simulink model "ADS"  (R2022a)
settings: Solver=VariableStepAuto  StartTime=0.0  StopTime=10.0  RelTol=1e-3
values from neighbouring files (symbols this model uses):
  GyroB = deg2rad(3/3600) * randn * ones(3,1)    [backend.m]
  T = 0.1    [ADS.m]    (also in backend.m)
undefined symbols (not defined in the file or in its folder): magnitude
libraries: commchan3 x1
settings Model: Creator=emmamarsden  LastModifiedBy=emmamarsden

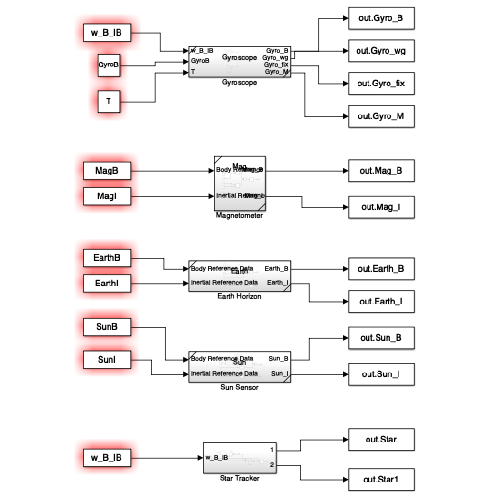
[thumbnail: Simulink's stored preview of the top-level diagram]
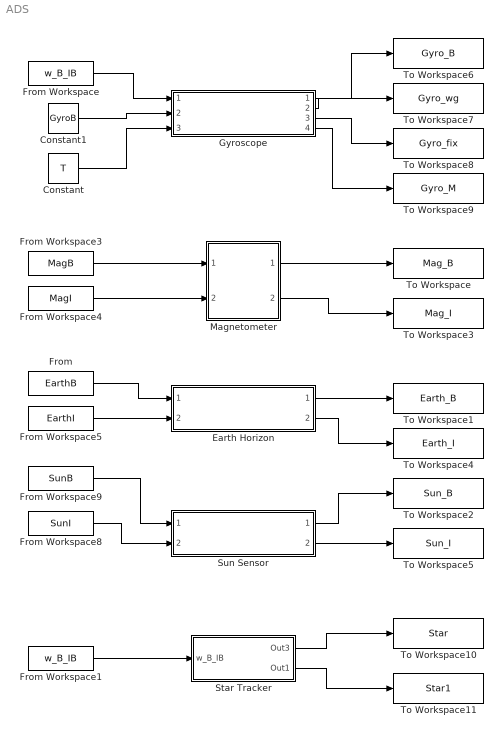
== system ADS ==
  Constant : Constant  Value=T
  Constant1 : Constant  Value=GyroB
  Earth Horizon : Subsystem  ReferencedSubsystem=Earth
  From : FromWorkspace  VariableName=EarthB  SampleTime=-1  ZeroCross=off
  From Workspace : FromWorkspace  VariableName=w_B_IB
  From Workspace1 : FromWorkspace  VariableName=w_B_IB
  From Workspace3 : FromWorkspace  VariableName=MagB
  From Workspace4 : FromWorkspace  VariableName=MagI
  From Workspace5 : FromWorkspace  VariableName=EarthI  ZeroCross=off
  From Workspace8 : FromWorkspace  VariableName=SunI
  From Workspace9 : FromWorkspace  VariableName=SunB
  Gyroscope : Subsystem  ReferencedSubsystem=Gyroscope
  Magnetometer : Subsystem  ReferencedSubsystem=Mag
  Star Tracker : Subsystem
  Sun Sensor : Subsystem  ReferencedSubsystem=Sun
  To Workspace : ToWorkspace  VariableName=Mag_B  SampleTime=-1
  To Workspace1 : ToWorkspace  VariableName=Earth_B  SampleTime=-1
  To Workspace10 : ToWorkspace  VariableName=Star  SaveFormat=Timeseries  SampleTime=-1
  To Workspace11 : ToWorkspace  VariableName=Star1  SaveFormat=Timeseries  SampleTime=-1
  To Workspace2 : ToWorkspace  VariableName=Sun_B  SaveFormat=Structure  SampleTime=-1
  To Workspace3 : ToWorkspace  VariableName=Mag_I  SampleTime=-1
  To Workspace4 : ToWorkspace  VariableName=Earth_I  SampleTime=-1
  To Workspace5 : ToWorkspace  VariableName=Sun_I  SaveFormat=Structure  SampleTime=-1
  To Workspace6 : ToWorkspace  VariableName=Gyro_B  SampleTime=-1
  To Workspace7 : ToWorkspace  VariableName=Gyro_wg  SampleTime=-1
  To Workspace8 : ToWorkspace  VariableName=Gyro_fix  SampleTime=-1
  To Workspace9 : ToWorkspace  VariableName=Gyro_M  SampleTime=-1
  wires:
  From Workspace5/1 -> Earth Horizon/2
  From Workspace4/1 -> Magnetometer/2
  From Workspace3/1 -> Magnetometer/1
  Magnetometer/1 -> To Workspace/1
  Magnetometer/2 -> To Workspace3/1
  Earth Horizon/1 -> To Workspace1/1
  Earth Horizon/2 -> To Workspace4/1
  From Workspace9/1 -> Sun Sensor/1
  From Workspace8/1 -> Sun Sensor/2
  From/1 -> Earth Horizon/1
  Sun Sensor/2 -> To Workspace5/1
  Sun Sensor/1 -> To Workspace2/1
  Constant1/1 -> Gyroscope/2
  From Workspace/1 -> Gyroscope/1
  Gyroscope/1 -> To Workspace6/1
  Gyroscope/2 -> To Workspace7/1
  Gyroscope/3 -> To Workspace8/1
  Gyroscope/4 -> To Workspace9/1
  Constant/1 -> Gyroscope/3
  From Workspace1/1 -> Star Tracker/1(w_B_IB)
  Star Tracker/1(Out3) -> To Workspace10/1
  Star Tracker/2(Out1) -> To Workspace11/1

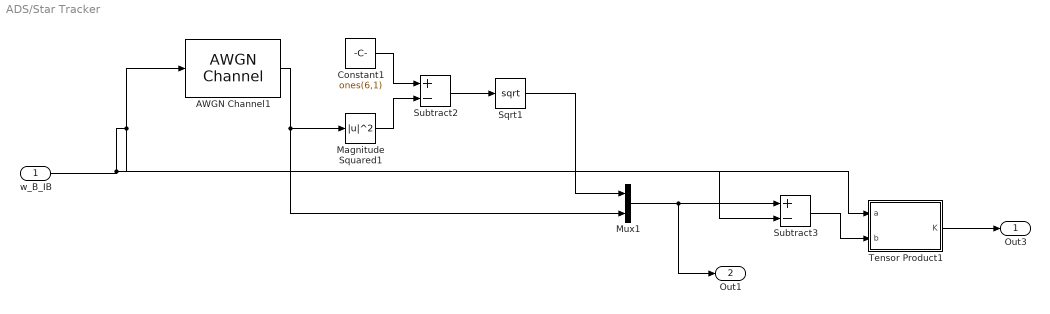
== system ADS/Star Tracker ==
  w_B_IB : Inport
  AWGN Channel1 : commchan3/AWGN Channel  InputProcessing=Columns as channels (frame based)  seed=67  noiseMode="Signal to noise ratio  (Eb/No)"  EbNodB=10  EsNodB=10  SNRdB=10  bitsPerSym=1  Ps=1  Tsym=1  variance=1
  Constant1 : Constant  Value=ones(6,1)
  Magnitude Squared1 : Math  Operator=magnitude^2
  Mux1 : Mux  Inputs=2
  Sqrt1 : Sqrt
  Subtract2 : Sum  Inputs=+-
  Subtract3 : Sum  Inputs=+-
  Tensor Product1 : MATLAB Function  TreatAsAtomicUnit=on
  Out3 : Outport
  Out1 : Outport  Port=2
  wires:
  w_B_IB/1 -> Tensor Product1/1(a), AWGN Channel1/1, Subtract3/2
  Tensor Product1/1(K) -> Out3/1
  Subtract3/1 -> Tensor Product1/2(b)
  Subtract2/1 -> Sqrt1/1
  Mux1/1 -> Out1/1, Subtract3/1
  AWGN Channel1/1 -> Magnitude Squared1/1, Mux1/2
  Sqrt1/1 -> Mux1/1
  Magnitude Squared1/1 -> Subtract2/2
  Constant1/1 -> Subtract2/1

== matlab function ADS/Star Tracker/Tensor Product1 ==
  data: a input; K output; b input
function K = fcn(a,b)

K = kron(a,b);
